simulink model "week2_inclass_longitudinalmodel_linear"  (R2020b)
settings: Solver=FixedStepAuto  StartTime=0.0  StopTime=5  RelTol=1e-3
undefined symbols (not defined in the file or in its folder): A, Cd, rho, v_0, vw_0
settings Model: Creator=anime  LastModifiedBy=anime

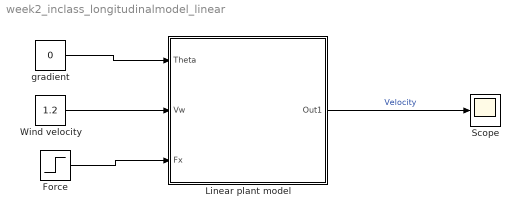
== system week2_inclass_longitudinalmodel_linear ==
  Force : Step  Time=3  SampleTime=0
  Linear plant model : Subsystem
  Scope : Scope
  Wind velocity : Constant  Value=1.2
  gradient : Constant  Value=0
  wires:
  Force/1 -> Linear plant model/3(Fx)
  Wind velocity/1 -> Linear plant model/2(Vw)
  Linear plant model/1(Out1) -> Scope/1  "Velocity"
  gradient/1 -> Linear plant model/1(Theta)

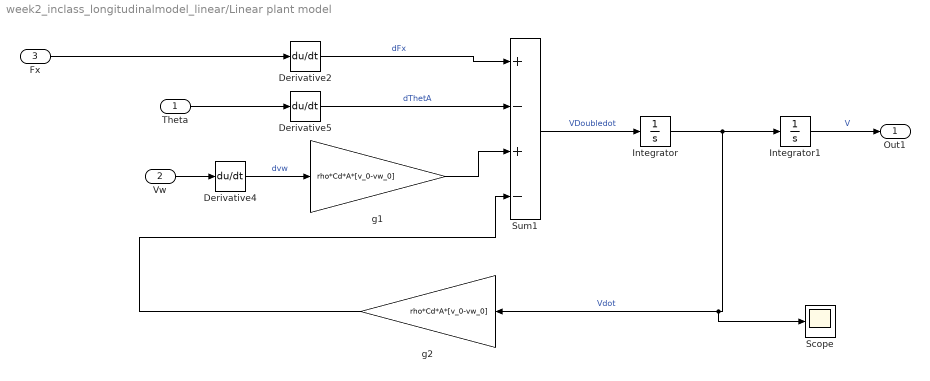
== system week2_inclass_longitudinalmodel_linear/Linear plant model ==
  Theta : Inport
  Vw : Inport  Port=2
  Fx : Inport  Port=3
  Derivative2 : Derivative
  Derivative4 : Derivative
  Derivative5 : Derivative
  Integrator : Integrator
  Integrator1 : Integrator
  Scope : Scope
  Sum1 : Sum  Inputs=+-+-
  g1 : Gain  Gain=rho*Cd*A*[v_0-vw_0]
  g2 : Gain  Gain=rho*Cd*A*[v_0-vw_0]
  Out1 : Outport
  wires:
  Derivative2/1 -> Sum1/1  "dFx"
  Vw/1 -> Derivative4/1
  Theta/1 -> Derivative5/1
  Derivative5/1 -> Sum1/2  "dThetA"
  Derivative4/1 -> g1/1  "dvw"
  g1/1 -> Sum1/3
  Sum1/1 -> Integrator/1  "VDoubledot"
  Integrator/1 -> Integrator1/1, Scope/1, g2/1  "Vdot"
  Integrator1/1 -> Out1/1  "V"
  g2/1 -> Sum1/4
  Fx/1 -> Derivative2/1
